simulink model "sampleModel541_pp_difftest"  (R2021a)
settings: Solver=VariableStepAuto  StartTime=0.0  StopTime=10.0  RelTol=1e-3
undefined symbols (not defined in the file): DiscIntNeverNeededParam, Newton, Raphson
libraries: simulink x23, pid_lib x5
settings Model: Creator=user  LastModifiedBy=user

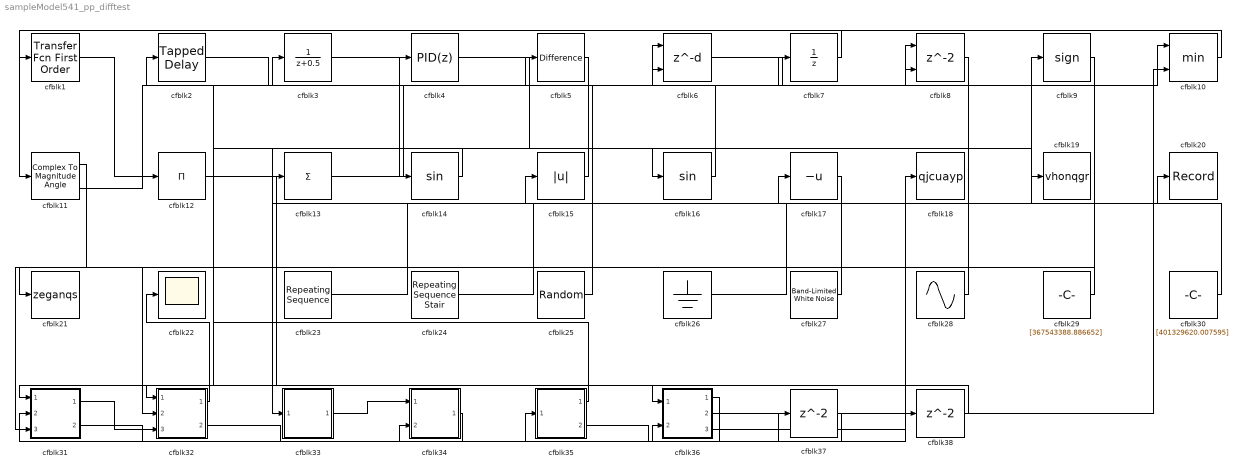
== system sampleModel541_pp_difftest ==
  cfblk1 : simulink/Discrete/Transfer Fcn First Order  PoleZ=0.95  ICPrevOutput=0.0  DoSatur=off
  cfblk10 : MinMax  Inputs=2
  cfblk11 : ComplexToMagnitudeAngle
  cfblk12 : Product  Inputs=*
  cfblk13 : Sum  Inputs=+
  cfblk14 : Trigonometry
  cfblk15 : Abs
  cfblk16 : Trigonometry
  cfblk17 : UnaryMinus
  cfblk18 : ToWorkspace  VariableName=qjcuayp  SaveFormat=Timeseries  SampleTime=-1
  cfblk19 : ToWorkspace  VariableName=vhonqgr  SaveFormat=Timeseries  SampleTime=-1
  cfblk2 : simulink/Discrete/Tapped Delay  vinit=0.0  samptime=-1  NumDelays=1  DelayOrder=Oldest  includeCurrent=off
  cfblk20 : Record  FileSettingsInternal="{\"entries\":[{\"content\":{\"excelSettings\":{\"content\":{},\"type\":\"Streamout.ExcelSettings\"}},\"type\":\"Streamout.FileSettingStorage\",\"uuid\":\"01edc3a3-d80d-4732-8608-4e9d142ed4ab\"}],\"packageUris\":[\"http://schema.mathworks.com/mf0/streamout_blocks/R2020a\"],\"version\":\"1.0\"}"  SignalsInternal="{\"entries\":[{\"content\":{\"signals\":[{\"content\":{\"blockPath\":[\"sampleModel541_pp_difftest/cfblk20\"],\"channel\":[],\"dimensions\":[1],\"domain\":\"samplemodel541_pp_difftest/cfblk20\",\"lineColor\":\"#7e2f8e\",\"plots\":[1],\"port\":1,\"sid\":[],\"signalID\":19,\"signalName\":\"cfblk24\"},\"type\":\"RecordBlkView.Signal\",\"uuid\":\"c9c95548-154d-48a7-8825-4786a1f0d84d\"}]},\"type\":\"RecordBlkView.InputSignals\",\"uuid\":\"a5788f2e-6ff7-4599-b457-e45010491cd0\"}],\"packageUris\":[\"http://schema.mathworks.com/mf0/streamout_blocks/R2020a\"],\"version\":\"1.0\"}"  VisualizationBindings="{\"sparklinesplugin\":{\"info\":[{\"bindingParametersList\":[],\"subplotID\":1}]}}"
  cfblk21 : ToWorkspace  VariableName=zeganqs  SaveFormat=Timeseries  SampleTime=-1
  cfblk22 : Scope
  cfblk23 : simulink/Sources/Repeating Sequence  rep_seq_t=[0 2]  rep_seq_y=[416477790.425688, 725633583.092416]
  cfblk24 : simulink/Sources/Repeating Sequence Stair  OutValues=[-702429095.453026, -136139678.587980]  tsamp=-1  OutMin=[]  OutMax=[]  OutDataTypeStr=double  OutputDataTypeScalingMode=double  OutDataType=fixdt(0,8)  ConRadixGroup=Best Precision: Vector-wise  OutScaling=2^-12
  cfblk25 : RandomNumber  Mean=[-5029.199072]  Variance=[76752.887216]  Seed=[360612598.000000]  SampleTime=0.1
  cfblk26 : Ground
  cfblk27 : simulink/Sources/Band-Limited White Noise  Cov=[8491605814.361879]  Ts=0.1  seed=[7568071354.000000]
  cfblk28 : Sin  Amplitude=[59962648.551395]  Bias=[-800425245.596998]  SampleTime=0
  cfblk29 : Constant  Value=[367543388.886652]  SampleTime=1
  cfblk3 : DiscreteTransferFcn  SampleTime=1
  cfblk30 : Constant  Value=[401329620.007595]  SampleTime=1
  cfblk31 : Subsystem
  cfblk32 : Subsystem
  cfblk33 : Subsystem
  cfblk34 : Subsystem
  cfblk35 : Subsystem
  cfblk36 : Subsystem
  cfblk37 : Delay  SampleTime=1
  cfblk38 : Delay  SampleTime=1
  cfblk4 : pid_lib/PID Controller  Controller=PID  Form=Parallel  TimeDomain=Discrete-time  UseExternalTs=off  SampleTime=1  IntegratorMethod=Forward Euler  FilterMethod=Forward Euler  ControllerParametersSource=internal  P=1  I=1  D=0  UseFilter=on  N=100  TunerSelectOption=Transfer Function Based (PID Tuner App)  InitialConditionSource=internal  InitialConditionForIntegrator=0  InitialConditionForFilter=0  DifferentiatorICPrevScaledInput=0  ExternalReset=none  TrackingMode=off  Kt=1  LimitOutput=off  SatLimitsSource=internal  UpperSaturationLimit=inf  LowerSaturationLimit=-inf  LinearizeAsGain=off  AntiWindupMode=none  Kb=1  POutMin=[]  POutMax=[]  IOutMin=[]  IOutMax=[]  DOutMin=[]  DOutMax=[]  NOutMin=[]  NOutMax=[]  SumOutMin=[]  SumOutMax=[]  SaturationOutMin=[]  SaturationOutMax=[]  PParamMin=[]  PParamMax=[]  IParamMin=[]  IParamMax=[]  DParamMin=[]  DParamMax=[]  NParamMin=[]  NParamMax=[]  KbParamMin=[]  KbParamMax=[]  KtParamMin=[]  KtParamMax=[]  KbOutMin=[]  KbOutMax=[]  KtOutMin=[]  KtOutMax=[]  IntegratorOutMin=[]  IntegratorOutMax=[]  FilterOutMin=[]  FilterOutMax=[]  SumI1OutMin=[]  SumI1OutMax=[]  SumI2OutMin=[]  SumI2OutMax=[]  SumI3OutMin=[]  SumI3OutMax=[]  SumI4OutMin=[]  SumI4OutMax=[]  SumDOutMin=[]  SumDOutMax=[]  DifferentiatorOutMin=[]  DifferentiatorOutMax=[]  FilterDiffOutCoefMin=[]  FilterDiffOutCoefMax=[]  ReciprocalOutMin=[]  ReciprocalOutMax=[]  SumDenOutMin=[]  SumDenOutMax=[]  SumNumOutMin=[]  SumNumOutMax=[]  DivideOutMin=[]  DivideOutMax=[]  UdiffTsProdOutMin=[]  UdiffTsProdOutMax=[]  NTsProdOutMin=[]  NTsProdOutMax=[]  UintegralTsProdOutMin=[]  UintegralTsProdOutMax=[]  UngainTsProdOutMin=[]  UngainTsProdOutMax=[]  IntegratorContinuousStateAttributes=''  IntegratorStateMustResolveToSignalObject=off  IntegratorRTWStateStorageClass=Auto  FilterContinuousStateAttributes=''  FilterStateMustResolveToSignalObject=off  FilterRTWStateStorageClass=Auto  ParallelPVariant=InternalParameters  IdealPVariant=Disabled  IVariant=InternalParameters  DVariant=InternalParameters  IntegratorVariant=Discrete  SatVariant=Disabled  AWVariant=Passthrough  PCopyVariant=Disabled  TRVariant=Disabled  FdbkBlocksVariant=Forward  IdealPFdbkVariant=Disabled  SatFdbkVariant=Disabled  DerivativeFilterVariant=ForwardEulerFilter  NVariant=InternalParameters  NCopyVariant=Disabled  FilterICVariant=InternalICsFilter  IntegratorICVariant=InternalICs  ExternalResetVariant=Disabled  TRSumVariant=Passthrough  SumFdbkVariant=Disabled  SumVariant=Sum_PID  TsampFilterVariant=InternalTs  TsampNgainVariant=Passthrough  TsampIntegralVariant=Passthrough  ExternalSaturationOutDataTypeStr=Inherit: Same as second input
  cfblk5 : simulink/Discrete/Difference  ICPrevInput=0.0  OutMin=[]  OutMax=[]  OutDataTypeStr=Inherit: Inherit via back propagation  OutDataType=fixdt(1, 16)  OutScaling=2^-10  DoSatur=off
  cfblk6 : Delay  DelayLengthSource=Input port  SampleTime=1
      settings: InputPortMap=u0,p1
  cfblk7 : UnitDelay  HasFrameUpgradeWarning=on
  cfblk8 : Delay  ShowEnablePort=on  SampleTime=1
      settings: InputPortMap=u0,e6
  cfblk9 : Signum
  wires:
  cfblk1/1 -> cfblk12/1
  cfblk10/1 -> cfblk11/1
  cfblk23/1 -> cfblk15/1
  cfblk24/1 -> cfblk20/1
  cfblk14/1 -> cfblk32/1(cfblk1)
  cfblk13/1 -> cfblk6/1
  cfblk35/1(cfblk2) -> cfblk2/1
  cfblk6/1 -> cfblk10/1
  cfblk3/1 -> cfblk14/1
  cfblk33/1(cfblk2) -> cfblk34/1(cfblk1)
  cfblk16/1 -> cfblk4/1
  cfblk5/1 -> cfblk33/1(cfblk1)
  cfblk26/1 -> cfblk9/1
  cfblk17/1 -> cfblk32/2(cfblk13)
  cfblk11/1 -> cfblk21/1
  cfblk32/1(cfblk2) -> cfblk22/1
  cfblk28/1 -> cfblk8/1
  cfblk29/1 -> cfblk7/1
  cfblk8/1 -> cfblk16/1
  cfblk12/1 -> cfblk36/1(cfblk1)
  cfblk7/1 -> cfblk1/1
  cfblk36/1(cfblk2) -> cfblk34/2(cfblk8)
  cfblk15/1 -> cfblk3/1
  cfblk27/1 -> cfblk13/1
  cfblk4/1 -> cfblk19/1
  cfblk2/1 -> cfblk6/2
  cfblk25/1 -> cfblk5/1
  cfblk30/1 -> cfblk17/1
  cfblk31/1(cfblk2) -> cfblk32/3(cfblk14)
  cfblk36/2(cfblk15) -> cfblk10/2
  cfblk31/2(cfblk12) -> cfblk35/1(cfblk1)
  cfblk34/1(cfblk2) -> cfblk31/2(cfblk10)
  cfblk9/1 -> cfblk31/3(cfblk11)
  cfblk11/2 -> cfblk8/2
  cfblk36/3(cfblk16) -> cfblk18/1
  cfblk32/2(cfblk15) -> cfblk37/1
  cfblk37/1 -> cfblk36/2(cfblk14)
  cfblk35/2(cfblk14) -> cfblk38/1
  cfblk38/1 -> cfblk31/1(cfblk1)

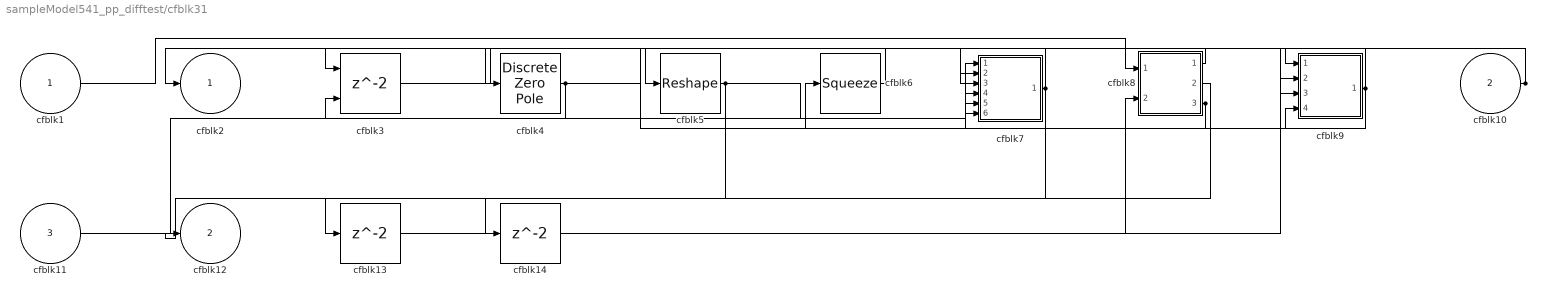
== system sampleModel541_pp_difftest/cfblk31 ==
  cfblk1 : Inport
  cfblk10 : Inport  Port=2
  cfblk11 : Inport  Port=3
  cfblk13 : Delay  SampleTime=1
  cfblk14 : Delay  SampleTime=1
  cfblk3 : Delay  ShowEnablePort=on  SampleTime=1
      settings: InputPortMap=u0,e6
  cfblk4 : DiscreteZeroPole  Poles=[0 0.5]  Gain=1
  cfblk5 : Reshape
  cfblk6 : Squeeze
  cfblk7 : Subsystem
  cfblk8 : Subsystem
  cfblk9 : Subsystem
  cfblk2 : Outport
  cfblk12 : Outport  Port=2
  wires:
  cfblk11/1 -> cfblk7/1(cfblk1)
  cfblk7/1(cfblk2) -> cfblk2/1, cfblk14/1
  cfblk1/1 -> cfblk8/1(cfblk1)
  cfblk8/1(cfblk2) -> cfblk3/1
  cfblk4/1 -> cfblk3/2, cfblk9/3(cfblk15), cfblk9/4(cfblk16)
  cfblk5/1 -> cfblk7/5(cfblk14), cfblk13/1
  cfblk8/2(cfblk14) -> cfblk12/1
  cfblk8/3(cfblk15) -> cfblk6/1, cfblk7/6(cfblk15)
  cfblk9/1(cfblk2) -> cfblk5/1, cfblk7/4(cfblk13)
  cfblk10/1 -> cfblk7/2(cfblk11), cfblk7/3(cfblk12)
  cfblk3/1 -> cfblk9/1(cfblk1)
  cfblk6/1 -> cfblk4/1
  cfblk13/1 -> cfblk8/2(cfblk13)
  cfblk14/1 -> cfblk9/2(cfblk14)

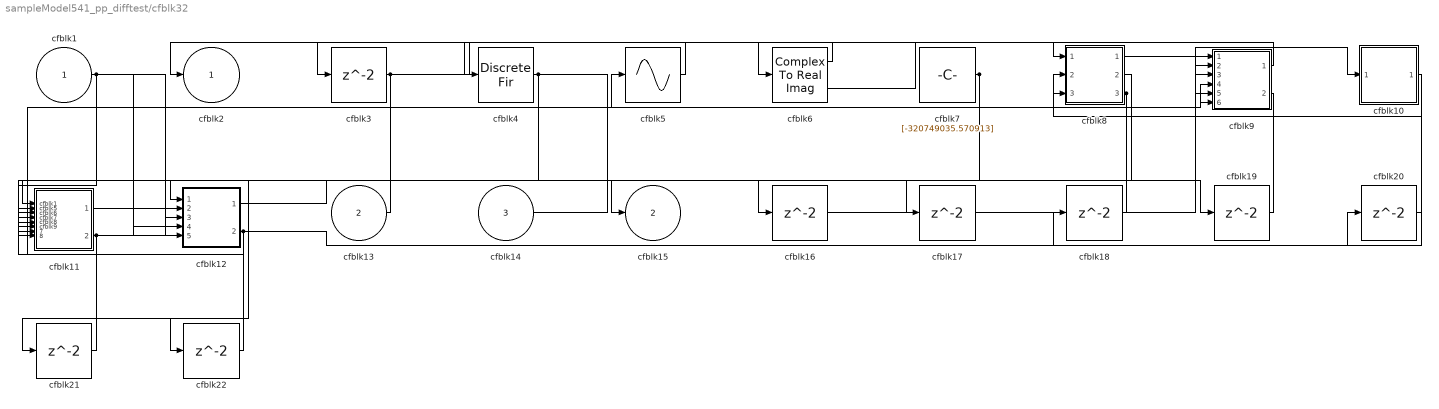
== system sampleModel541_pp_difftest/cfblk32 ==
  cfblk1 : Inport
  cfblk13 : Inport  Port=2
  cfblk14 : Inport  Port=3
  cfblk10 : Subsystem
  cfblk11 : Subsystem
  cfblk12 : Subsystem
  cfblk{3,16..22} (8 alike) : Delay  SampleTime=1
  cfblk4 : DiscreteFir  SampleTime=1
  cfblk5 : Sin  TimeSource=Use external signal  SampleTime=0
  cfblk6 : ComplexToRealImag
  cfblk7 : Constant  Value=[-320749035.570913]  SampleTime=1
  cfblk8 : Subsystem
  cfblk9 : Subsystem
  cfblk2 : Outport
  cfblk15 : Outport  Port=2
  wires:
  cfblk7/1 -> cfblk15/1, cfblk11/2(cfblk5)
  cfblk3/1 -> cfblk6/1, cfblk11/3(cfblk6), cfblk11/5(cfblk8)
  cfblk4/1 -> cfblk11/4(cfblk7), cfblk16/1
  cfblk5/1 -> cfblk2/1
  cfblk11/2(cfblk12) -> cfblk5/1, cfblk8/3(cfblk7)
  cfblk14/1 -> cfblk9/4(cfblk14)
  cfblk12/2(cfblk12) -> cfblk20/1, cfblk21/1
  cfblk1/1 -> cfblk9/6(cfblk16), cfblk12/4(cfblk10), cfblk12/5(cfblk11), cfblk11/8(cfblk11)
  cfblk6/1 -> cfblk4/1
  cfblk6/2 -> cfblk8/1(cfblk1)
  cfblk8/1(cfblk2) -> cfblk10/1(cfblk1)
  cfblk13/1 -> cfblk12/1(cfblk1)
  cfblk9/1(cfblk2) -> cfblk3/1
  cfblk9/2(cfblk17) -> cfblk8/2(cfblk6)
  cfblk8/2(cfblk8) -> cfblk12/2(cfblk8)
  cfblk8/3(cfblk9) -> cfblk12/3(cfblk9), cfblk22/1
  cfblk16/1 -> cfblk9/1(cfblk1)
  cfblk11/1(cfblk2) -> cfblk17/1
  cfblk17/1 -> cfblk9/2(cfblk12)
  cfblk10/1(cfblk2) -> cfblk18/1
  cfblk18/1 -> cfblk11/1(cfblk1)
  cfblk12/1(cfblk2) -> cfblk19/1
  cfblk19/1 -> cfblk9/3(cfblk13)
  cfblk20/1 -> cfblk9/5(cfblk15)
  cfblk21/1 -> cfblk11/7(cfblk10)
  cfblk22/1 -> cfblk11/6(cfblk9)

== system sampleModel541_pp_difftest/cfblk33 ==
  cfblk1 : Inport
  cfblk10 : Delay  SampleTime=1
  cfblk3 : Product  Inputs=*
  cfblk4 : Signum
  cfblk5 : Subsystem
  cfblk6 : Subsystem
  cfblk7 : Subsystem
  cfblk8 : Delay  SampleTime=1
  cfblk9 : Delay  SampleTime=1
  cfblk2 : Outport
  wires:
  cfblk6/1(cfblk2) -> cfblk4/1
  cfblk1/1 -> cfblk2/1
  cfblk3/1 -> cfblk5/2(cfblk8)
  cfblk5/1(cfblk2) -> cfblk6/2(cfblk9)
  cfblk5/2(cfblk9) -> cfblk7/1(cfblk1)
  cfblk4/1 -> cfblk8/1
  cfblk8/1 -> cfblk6/1(cfblk1)
  cfblk7/1(cfblk2) -> cfblk9/1
  cfblk9/1 -> cfblk5/1(cfblk1)
  cfblk7/2(cfblk7) -> cfblk10/1
  cfblk10/1 -> cfblk3/1

== system sampleModel541_pp_difftest/cfblk34 ==
  cfblk1 : Inport
  cfblk8 : Inport  Port=2
  cfblk{9..14} (6 alike) : Delay  SampleTime=1
  cfblk3 : simulink/Discrete/Tapped Delay  vinit=0.0  samptime=-1  NumDelays=1  DelayOrder=Oldest  includeCurrent=off
  cfblk4 : Product
  cfblk5 : Product
  cfblk6 : Sum  Inputs=+-
  cfblk7 : Subsystem
  cfblk2 : Outport
  wires:
  cfblk4/1 -> cfblk3/1, cfblk13/1
  cfblk8/1 -> cfblk6/1
  cfblk1/1 -> cfblk2/1, cfblk7/4(cfblk14)
  cfblk5/1 -> cfblk9/1, cfblk10/1, cfblk11/1
  cfblk7/1(cfblk2) -> cfblk6/2
  cfblk3/1 -> cfblk5/1, cfblk12/1
  cfblk6/1 -> cfblk4/2, cfblk14/1
  cfblk7/2(cfblk17) -> cfblk5/2
  cfblk9/1 -> cfblk4/1
  cfblk10/1 -> cfblk7/2(cfblk12)
  cfblk11/1 -> cfblk7/3(cfblk13)
  cfblk12/1 -> cfblk7/1(cfblk1)
  cfblk13/1 -> cfblk7/5(cfblk15)
  cfblk14/1 -> cfblk7/6(cfblk16)

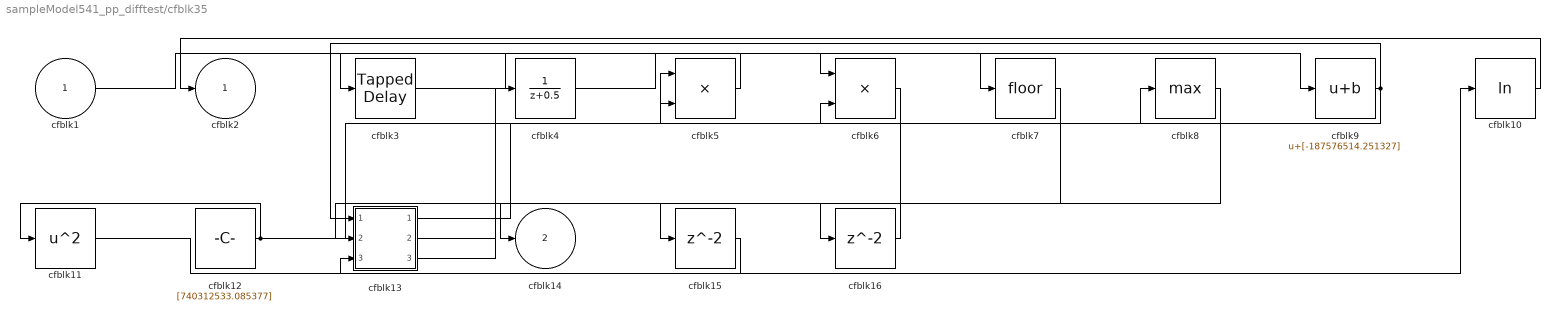
== system sampleModel541_pp_difftest/cfblk35 ==
  cfblk1 : Inport
  cfblk10 : Math  Operator=log  SaturateOnIntegerOverflow=on
  cfblk11 : Math  Operator=square  SaturateOnIntegerOverflow=on
  cfblk12 : Constant  Value=[740312533.085377]  SampleTime=1
  cfblk13 : Subsystem
  cfblk15 : Delay  SampleTime=1
  cfblk16 : Delay  SampleTime=1
  cfblk3 : simulink/Discrete/Tapped Delay  vinit=0.0  samptime=-1  NumDelays=1  DelayOrder=Oldest  includeCurrent=off
  cfblk4 : DiscreteTransferFcn  SampleTime=1
  cfblk5 : Product  Inputs=**
  cfblk6 : Product  Inputs=**
  cfblk7 : Rounding
  cfblk8 : MinMax  Function=max
  cfblk9 : Bias  Bias=[-187576514.251327]
  cfblk2 : Outport
  cfblk14 : Outport  Port=2
  wires:
  cfblk5/1 -> cfblk3/1
  cfblk12/1 -> cfblk5/1, cfblk11/1
  cfblk9/1 -> cfblk13/1(cfblk1), cfblk6/2
  cfblk11/1 -> cfblk10/1
  cfblk3/1 -> cfblk7/1
  cfblk13/1(cfblk2) -> cfblk5/2
  cfblk10/1 -> cfblk2/1
  cfblk1/1 -> cfblk9/1
  cfblk8/1 -> cfblk14/1
  cfblk4/1 -> cfblk6/1
  cfblk13/2(cfblk12) -> cfblk8/1
  cfblk13/3(cfblk13) -> cfblk4/1
  cfblk7/1 -> cfblk15/1
  cfblk15/1 -> cfblk13/3(cfblk11)
  cfblk6/1 -> cfblk16/1
  cfblk16/1 -> cfblk13/2(cfblk10)

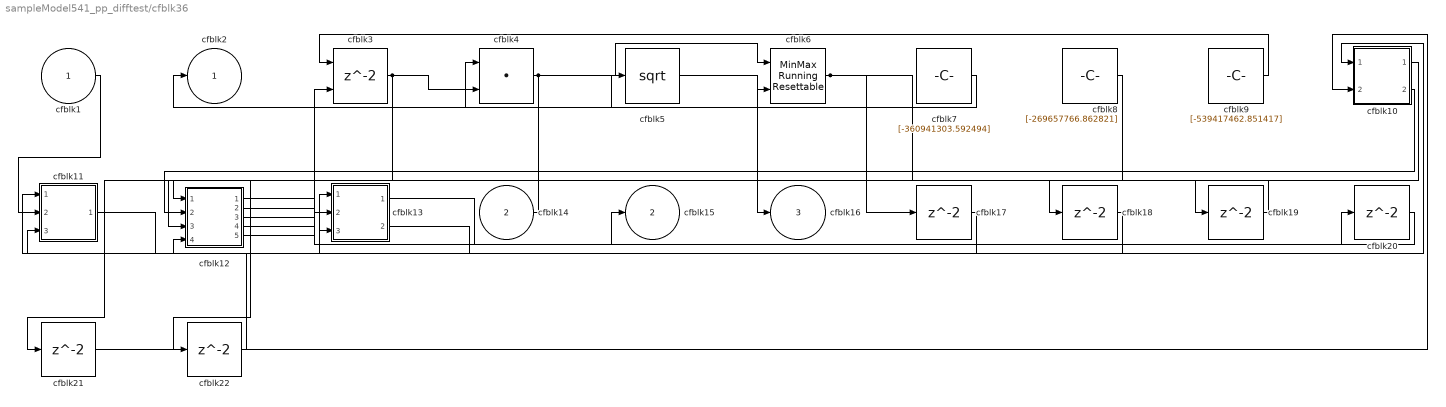
== system sampleModel541_pp_difftest/cfblk36 ==
  cfblk1 : Inport
  cfblk14 : Inport  Port=2
  cfblk10 : Subsystem
  cfblk11 : Subsystem
  cfblk12 : Subsystem
  cfblk13 : Subsystem
  cfblk{17..22} (6 alike) : Delay  SampleTime=1
  cfblk3 : Delay  ShowEnablePort=on  SampleTime=1
      settings: InputPortMap=u0,e6
  cfblk4 : DotProduct  InputSameDT=on  OutDataTypeStr=Inherit: Inherit via internal rule
  cfblk5 : Sqrt  SaturateOnIntegerOverflow=on
  cfblk6 : simulink/Math Operations/MinMax Running Resettable  Function=min  vinit=0.0
  cfblk7 : Constant  Value=[-360941303.592494]  SampleTime=1
  cfblk8 : Constant  Value=[-269657766.862821]  SampleTime=1
  cfblk9 : Constant  Value=[-539417462.851417]  SampleTime=1
  cfblk2 : Outport
  cfblk15 : Outport  Port=2
  cfblk16 : Outport  Port=3
  wires:
  cfblk10/1(cfblk2) -> cfblk12/1(cfblk1)
  cfblk4/1 -> cfblk6/1, cfblk21/1
  cfblk7/1 -> cfblk5/1
  cfblk10/2(cfblk8) -> cfblk12/2(cfblk8)
  cfblk3/1 -> cfblk4/2, cfblk22/1
  cfblk14/1 -> cfblk2/1
  cfblk9/1 -> cfblk3/1
  cfblk8/1 -> cfblk12/3(cfblk9)
  cfblk5/1 -> cfblk16/1
  cfblk11/1(cfblk2) -> cfblk13/1(cfblk1)
  cfblk13/1(cfblk2) -> cfblk15/1
  cfblk6/1 -> cfblk17/1, cfblk18/1
  cfblk12/1(cfblk2) -> cfblk6/2
  cfblk1/1 -> cfblk11/2(cfblk6)
  cfblk13/2(cfblk16) -> cfblk10/1(cfblk1)
  cfblk12/4(cfblk13) -> cfblk4/1
  cfblk12/5(cfblk14) -> cfblk3/2
  cfblk17/1 -> cfblk12/4(cfblk10)
  cfblk18/1 -> cfblk11/3(cfblk7)
  cfblk12/2(cfblk11) -> cfblk19/1
  cfblk19/1 -> cfblk13/2(cfblk14)
  cfblk12/3(cfblk12) -> cfblk20/1
  cfblk20/1 -> cfblk13/3(cfblk15)
  cfblk21/1 -> cfblk10/2(cfblk7)
  cfblk22/1 -> cfblk11/1(cfblk1)

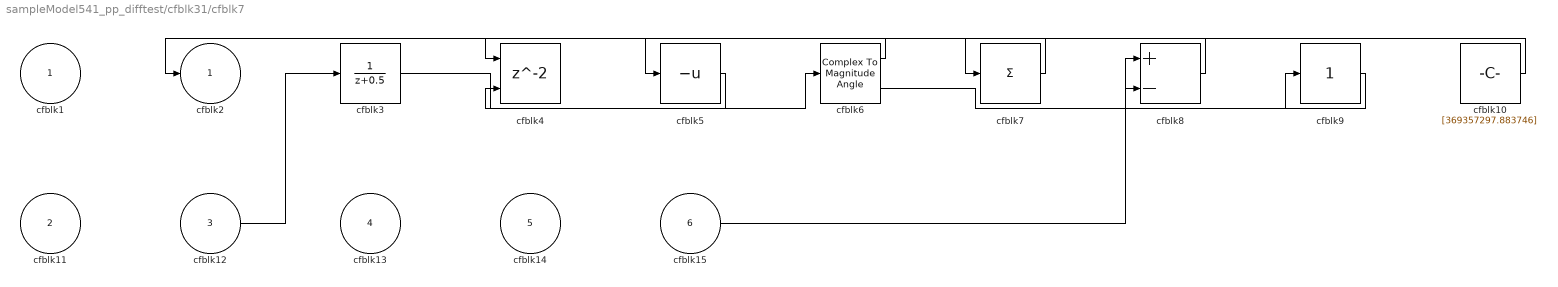
== system sampleModel541_pp_difftest/cfblk31/cfblk7 ==
  cfblk1 : Inport
  cfblk11 : Inport  Port=2
  cfblk12 : Inport  Port=3
  cfblk13 : Inport  Port=4
  cfblk14 : Inport  Port=5
  cfblk15 : Inport  Port=6
  cfblk10 : Constant  Value=[369357297.883746]  SampleTime=1
  cfblk3 : DiscreteTransferFcn  SampleTime=1
  cfblk4 : Delay  ShowEnablePort=on  SampleTime=1
      settings: InputPortMap=u0,e6
  cfblk5 : UnaryMinus
  cfblk6 : ComplexToMagnitudeAngle
  cfblk7 : Sum  Inputs=+
  cfblk8 : Sum  Inputs=+-
  cfblk9 : simulink/Math Operations/Slider Gain  gain=1  low=0  high=2
  cfblk2 : Outport
  wires:
  cfblk6/1 -> cfblk2/1
  cfblk6/2 -> cfblk9/1
  cfblk8/1 -> cfblk7/1
  cfblk7/1 -> cfblk5/1
  cfblk3/1 -> cfblk6/1
  cfblk10/1 -> cfblk4/1
  cfblk15/1 -> cfblk8/1
  cfblk12/1 -> cfblk3/1
  cfblk5/1 -> cfblk4/2
  cfblk9/1 -> cfblk8/2

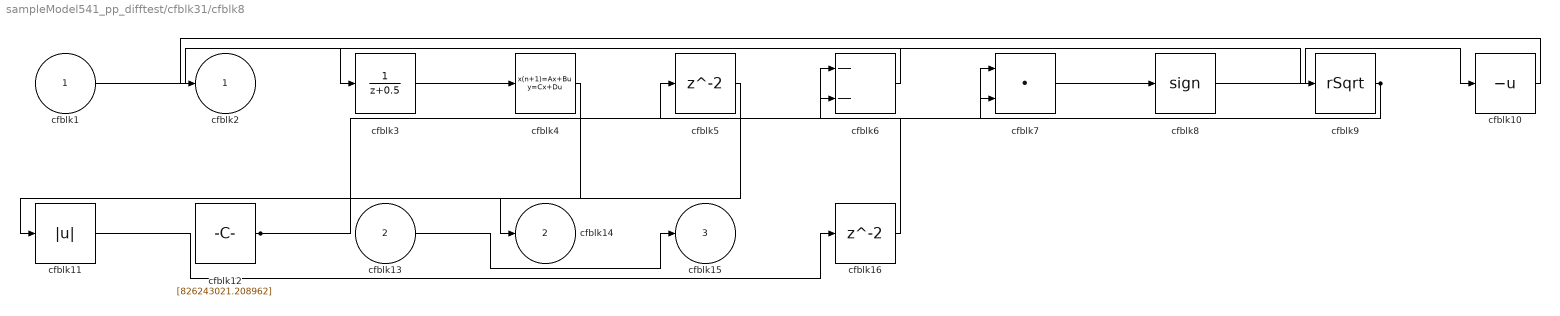
== system sampleModel541_pp_difftest/cfblk31/cfblk8 ==
  cfblk1 : Inport
  cfblk13 : Inport  Port=2
  cfblk10 : UnaryMinus
  cfblk11 : Abs
  cfblk12 : Constant  Value=[826243021.208962]  SampleTime=1
  cfblk16 : Delay  SampleTime=1
  cfblk3 : DiscreteTransferFcn  SampleTime=1
  cfblk4 : DiscreteStateSpace
  cfblk5 : Delay  SampleTime=1
  cfblk6 : Sum  Inputs=--
  cfblk7 : DotProduct  InputSameDT=on  OutDataTypeStr=Inherit: Inherit via internal rule
  cfblk8 : Signum
  cfblk9 : Sqrt  Operator=rSqrt  AlgorithmType=Newton-Raphson  SaturateOnIntegerOverflow=on
  cfblk2 : Outport
  cfblk14 : Outport  Port=2
  cfblk15 : Outport  Port=3
  wires:
  cfblk8/1 -> cfblk10/1
  cfblk4/1 -> cfblk14/1
  cfblk3/1 -> cfblk4/1
  cfblk9/1 -> cfblk6/1, cfblk7/2
  cfblk1/1 -> cfblk9/1
  cfblk12/1 -> cfblk6/2, cfblk7/1
  cfblk13/1 -> cfblk15/1
  cfblk7/1 -> cfblk8/1
  cfblk6/1 -> cfblk3/1
  cfblk5/1 -> cfblk11/1
  cfblk10/1 -> cfblk2/1
  cfblk11/1 -> cfblk16/1
  cfblk16/1 -> cfblk5/1

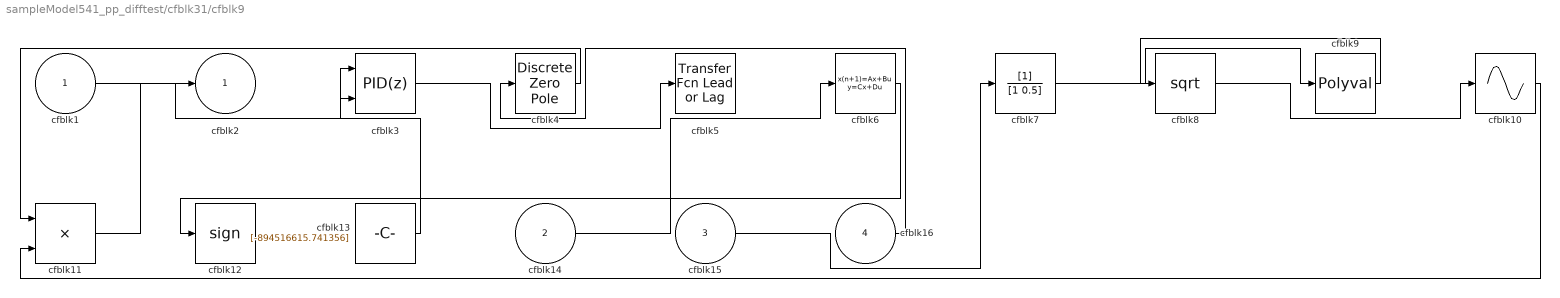
== system sampleModel541_pp_difftest/cfblk31/cfblk9 ==
  cfblk1 : Inport
  cfblk14 : Inport  Port=2
  cfblk15 : Inport  Port=3
  cfblk16 : Inport  Port=4
  cfblk10 : Sin  TimeSource=Use external signal  SampleTime=0
  cfblk11 : Product  Inputs=**
  cfblk12 : Signum
  cfblk13 : Constant  Value=[-894516615.741356]  SampleTime=1
  cfblk3 : pid_lib/PID Controller (2DOF)  Controller=PID  Form=Parallel  TimeDomain=Discrete-time  UseExternalTs=off  SampleTime=1  IntegratorMethod=Forward Euler  FilterMethod=Forward Euler  ControllerParametersSource=internal  P=1  I=1  D=0  UseFilter=on  N=100  b=1  c=1  TunerSelectOption=Transfer Function Based (PID Tuner App)  InitialConditionSource=internal  InitialConditionForIntegrator=0  InitialConditionForFilter=0  DifferentiatorICPrevScaledInput=0  ExternalReset=none  TrackingMode=off  Kt=1  LimitOutput=off  SatLimitsSource=internal  UpperSaturationLimit=inf  LowerSaturationLimit=-inf  LinearizeAsGain=off  AntiWindupMode=none  Kb=1  POutMin=[]  POutMax=[]  IOutMin=[]  IOutMax=[]  DOutMin=[]  DOutMax=[]  NOutMin=[]  NOutMax=[]  bOutMin=[]  bOutMax=[]  cOutMin=[]  cOutMax=[]  SumOutMin=[]  SumOutMax=[]  SaturationOutMin=[]  SaturationOutMax=[]  PParamMin=[]  PParamMax=[]  IParamMin=[]  IParamMax=[]  DParamMin=[]  DParamMax=[]  NParamMin=[]  NParamMax=[]  bParamMin=[]  bParamMax=[]  cParamMin=[]  cParamMax=[]  KbParamMin=[]  KbParamMax=[]  KtParamMin=[]  KtParamMax=[]  KbOutMin=[]  KbOutMax=[]  KtOutMin=[]  KtOutMax=[]  IntegratorOutMin=[]  IntegratorOutMax=[]  FilterOutMin=[]  FilterOutMax=[]  SumI1OutMin=[]  SumI1OutMax=[]  SumI2OutMin=[]  SumI2OutMax=[]  SumI3OutMin=[]  SumI3OutMax=[]  SumI4OutMin=[]  SumI4OutMax=[]  SumDOutMin=[]  SumDOutMax=[]  Sum1OutMin=[]  Sum1OutMax=[]  Sum2OutMin=[]  Sum2OutMax=[]  Sum3OutMin=[]  Sum3OutMax=[]  DifferentiatorOutMin=[]  DifferentiatorOutMax=[]  FilterDiffOutCoefMin=[]  FilterDiffOutCoefMax=[]  ReciprocalOutMin=[]  ReciprocalOutMax=[]  SumDenOutMin=[]  SumDenOutMax=[]  SumNumOutMin=[]  SumNumOutMax=[]  DivideOutMin=[]  DivideOutMax=[]  UdiffTsProdOutMin=[]  UdiffTsProdOutMax=[]  NTsProdOutMin=[]  NTsProdOutMax=[]  UintegralTsProdOutMin=[]  UintegralTsProdOutMax=[]  UngainTsProdOutMin=[]  UngainTsProdOutMax=[]  IntegratorContinuousStateAttributes=''  IntegratorStateMustResolveToSignalObject=off  IntegratorRTWStateStorageClass=Auto  FilterContinuousStateAttributes=''  FilterStateMustResolveToSignalObject=off  FilterRTWStateStorageClass=Auto  ParallelPVariant=InternalParameters  IdealPVariant=Disabled  IVariant=InternalParameters  DVariant=InternalParameters  bVariant=InternalParameters  cVariant=InternalParameters  IntegratorVariant=Discrete  SatVariant=Disabled  AWVariant=Passthrough  PCopyVariant=Disabled  TRVariant=Disabled  FdbkBlocksVariant=Forward  IdealPFdbkVariant=Disabled  SatFdbkVariant=Disabled  DerivativeFilterVariant=ForwardEulerFilter  NVariant=InternalParameters  NCopyVariant=Disabled  FilterICVariant=InternalICsFilter  IntegratorICVariant=InternalICs  ExternalResetVariant=Disabled  TRSumVariant=Passthrough  SumFdbkVariant=Disabled  SumVariant=Sum_PID  TsampFilterVariant=InternalTs  TsampNgainVariant=Passthrough  TsampIntegralVariant=Passthrough  ExternalSaturationOutDataTypeStr=Inherit: Same as second input
      settings: SourceProductBaseCode=SL
  cfblk4 : DiscreteZeroPole  Poles=[0 0.5]  Gain=1
  cfblk5 : simulink/Discrete/Transfer Fcn Lead or Lag  PoleZ=0.95  ZeroZ=0.75  ICPrevOutput=0.0  ICPrevInput=0.0  DoSatur=off
      settings: SourceProductBaseCode=SL
  cfblk6 : DiscreteStateSpace
  cfblk7 : DiscreteFilter  SampleTime=1
  cfblk8 : Sqrt  SaturateOnIntegerOverflow=on
  cfblk9 : Polyval  Coefs=[ +2.081618890e-019, -1.441693666e-014, +4.719686976e-010, -8.536869453e-006, +1.621573104e-001, -8.087801117e+001 ]
  cfblk2 : Outport
  wires:
  cfblk6/1 -> cfblk12/1
  cfblk11/1 -> cfblk2/1
  cfblk13/1 -> cfblk3/1
  cfblk14/1 -> cfblk6/1
  cfblk4/1 -> cfblk11/1
  cfblk7/1 -> cfblk9/1
  cfblk15/1 -> cfblk7/1
  cfblk8/1 -> cfblk10/1
  cfblk10/1 -> cfblk11/2
  cfblk9/1 -> cfblk8/1
  cfblk1/1 -> cfblk3/2
  cfblk16/1 -> cfblk4/1
  cfblk3/1 -> cfblk5/1

== system sampleModel541_pp_difftest/cfblk32/cfblk10 ==
  cfblk1 : Inport
  cfblk3 : DiscreteFir  SampleTime=1
  cfblk4 : Product  Inputs=*
  cfblk5 : Squeeze
  cfblk6 : Product  Inputs=**
  cfblk7 : Math  SaturateOnIntegerOverflow=on
  cfblk2 : Outport
  wires:
  cfblk6/1 -> cfblk2/1
  cfblk3/1 -> cfblk6/1
  cfblk1/1 -> cfblk4/1
  cfblk7/1 -> cfblk5/1
  cfblk4/1 -> cfblk7/1, cfblk3/1
  cfblk5/1 -> cfblk6/2

== system sampleModel541_pp_difftest/cfblk32/cfblk11 ==
  cfblk1 : Inport
  cfblk5 : Inport  Port=2
  cfblk6 : Inport  Port=3
  cfblk7 : Inport  Port=4
  cfblk8 : Inport  Port=5
  cfblk9 : Inport  Port=6
  cfblk10 : Inport  Port=7
  cfblk11 : Inport  Port=8
  cfblk3 : simulink/Discrete/Difference  ICPrevInput=0.0  OutMin=[]  OutMax=[]  OutDataTypeStr=Inherit: Inherit via back propagation  OutDataType=fixdt(1, 16)  OutScaling=2^-10  DoSatur=off
  cfblk4 : Polyval  Coefs=[ +2.081618890e-019, -1.441693666e-014, +4.719686976e-010, -8.536869453e-006, +1.621573104e-001, -8.087801117e+001 ]
  cfblk2 : Outport
  cfblk12 : Outport  Port=2
  wires:
  cfblk9/1 -> cfblk2/1
  cfblk3/1 -> cfblk12/1
  cfblk7/1 -> cfblk4/1
  cfblk4/1 -> cfblk3/1

== system sampleModel541_pp_difftest/cfblk32/cfblk12 ==
  cfblk1 : Inport
  cfblk8 : Inport  Port=2
  cfblk9 : Inport  Port=3
  cfblk10 : Inport  Port=4
  cfblk11 : Inport  Port=5
  cfblk3 : DiscreteTransferFcn  SampleTime=1
  cfblk4 : DiscreteTransferFcn  SampleTime=1
  cfblk5 : ComplexToRealImag
  cfblk6 : Abs
  cfblk7 : Sum  Inputs=+
  cfblk2 : Outport
  cfblk12 : Outport  Port=2
  wires:
  cfblk1/1 -> cfblk7/1
  cfblk7/1 -> cfblk12/1
  cfblk9/1 -> cfblk5/1
  cfblk3/1 -> cfblk2/1
  cfblk5/1 -> cfblk3/1
  cfblk5/2 -> cfblk6/1
  cfblk10/1 -> cfblk4/1

== system sampleModel541_pp_difftest/cfblk32/cfblk8 ==
  cfblk1 : Inport
  cfblk6 : Inport  Port=2
  cfblk7 : Inport  Port=3
  cfblk10 : Delay  SampleTime=1
  cfblk3 : DiscreteFilter  SampleTime=1
  cfblk4 : DiscreteZeroPole  Poles=[0 0.5]  Gain=1
  cfblk5 : Product
  cfblk2 : Outport
  cfblk8 : Outport  Port=2
  cfblk9 : Outport  Port=3
  wires:
  cfblk6/1 -> cfblk8/1
  cfblk1/1 -> cfblk9/1
  cfblk5/1 -> cfblk2/1, cfblk10/1
  cfblk3/1 -> cfblk4/1
  cfblk4/1 -> cfblk5/1
  cfblk7/1 -> cfblk5/2
  cfblk10/1 -> cfblk3/1

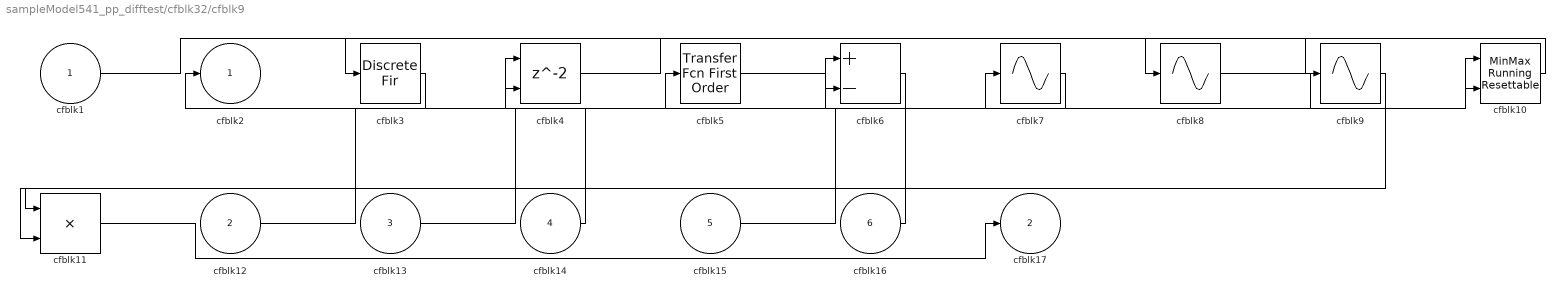
== system sampleModel541_pp_difftest/cfblk32/cfblk9 ==
  cfblk1 : Inport
  cfblk12 : Inport  Port=2
  cfblk13 : Inport  Port=3
  cfblk14 : Inport  Port=4
  cfblk15 : Inport  Port=5
  cfblk16 : Inport  Port=6
  cfblk10 : simulink/Math Operations/MinMax Running Resettable  Function=min  vinit=0.0
  cfblk11 : Product
  cfblk3 : DiscreteFir  SampleTime=1
  cfblk4 : Delay  ShowEnablePort=on  SampleTime=1
      settings: InputPortMap=u0,e6
  cfblk5 : simulink/Discrete/Transfer Fcn First Order  PoleZ=0.95  ICPrevOutput=0.0  DoSatur=off
  cfblk6 : Sum  Inputs=+-
  cfblk7 : Sin  TimeSource=Use external signal  SampleTime=0
  cfblk8 : Sin  TimeSource=Use external signal  SampleTime=0
  cfblk9 : Sin  TimeSource=Use external signal  SampleTime=0
  cfblk2 : Outport
  cfblk17 : Outport  Port=2
  wires:
  cfblk16/1 -> cfblk5/1
  cfblk11/1 -> cfblk17/1
  cfblk10/1 -> cfblk3/1
  cfblk6/1 -> cfblk11/1
  cfblk15/1 -> cfblk10/1
  cfblk9/1 -> cfblk11/2
  cfblk4/1 -> cfblk8/1
  cfblk8/1 -> cfblk10/2
  cfblk14/1 -> cfblk4/1
  cfblk3/1 -> cfblk2/1
  cfblk1/1 -> cfblk9/1
  cfblk13/1 -> cfblk7/1
  cfblk12/1 -> cfblk6/1
  cfblk7/1 -> cfblk4/2
  cfblk5/1 -> cfblk6/2

== system sampleModel541_pp_difftest/cfblk33/cfblk5 ==
  cfblk1 : Inport
  cfblk8 : Inport  Port=2
  cfblk3 : UnitDelay  HasFrameUpgradeWarning=on
  cfblk4 : pid_lib/PID Controller  Controller=PID  Form=Parallel  TimeDomain=Discrete-time  UseExternalTs=off  SampleTime=1  IntegratorMethod=Forward Euler  FilterMethod=Forward Euler  ControllerParametersSource=internal  P=1  I=1  D=0  UseFilter=on  N=100  TunerSelectOption=Transfer Function Based (PID Tuner App)  InitialConditionSource=internal  InitialConditionForIntegrator=0  InitialConditionForFilter=0  DifferentiatorICPrevScaledInput=0  ExternalReset=none  TrackingMode=off  Kt=1  LimitOutput=off  SatLimitsSource=internal  UpperSaturationLimit=inf  LowerSaturationLimit=-inf  LinearizeAsGain=off  AntiWindupMode=none  Kb=1  POutMin=[]  POutMax=[]  IOutMin=[]  IOutMax=[]  DOutMin=[]  DOutMax=[]  NOutMin=[]  NOutMax=[]  SumOutMin=[]  SumOutMax=[]  SaturationOutMin=[]  SaturationOutMax=[]  PParamMin=[]  PParamMax=[]  IParamMin=[]  IParamMax=[]  DParamMin=[]  DParamMax=[]  NParamMin=[]  NParamMax=[]  KbParamMin=[]  KbParamMax=[]  KtParamMin=[]  KtParamMax=[]  KbOutMin=[]  KbOutMax=[]  KtOutMin=[]  KtOutMax=[]  IntegratorOutMin=[]  IntegratorOutMax=[]  FilterOutMin=[]  FilterOutMax=[]  SumI1OutMin=[]  SumI1OutMax=[]  SumI2OutMin=[]  SumI2OutMax=[]  SumI3OutMin=[]  SumI3OutMax=[]  SumI4OutMin=[]  SumI4OutMax=[]  SumDOutMin=[]  SumDOutMax=[]  DifferentiatorOutMin=[]  DifferentiatorOutMax=[]  FilterDiffOutCoefMin=[]  FilterDiffOutCoefMax=[]  ReciprocalOutMin=[]  ReciprocalOutMax=[]  SumDenOutMin=[]  SumDenOutMax=[]  SumNumOutMin=[]  SumNumOutMax=[]  DivideOutMin=[]  DivideOutMax=[]  UdiffTsProdOutMin=[]  UdiffTsProdOutMax=[]  NTsProdOutMin=[]  NTsProdOutMax=[]  UintegralTsProdOutMin=[]  UintegralTsProdOutMax=[]  UngainTsProdOutMin=[]  UngainTsProdOutMax=[]  IntegratorContinuousStateAttributes=''  IntegratorStateMustResolveToSignalObject=off  IntegratorRTWStateStorageClass=Auto  FilterContinuousStateAttributes=''  FilterStateMustResolveToSignalObject=off  FilterRTWStateStorageClass=Auto  ParallelPVariant=InternalParameters  IdealPVariant=Disabled  IVariant=InternalParameters  DVariant=InternalParameters  IntegratorVariant=Discrete  SatVariant=Disabled  AWVariant=Passthrough  PCopyVariant=Disabled  TRVariant=Disabled  FdbkBlocksVariant=Forward  IdealPFdbkVariant=Disabled  SatFdbkVariant=Disabled  DerivativeFilterVariant=ForwardEulerFilter  NVariant=InternalParameters  NCopyVariant=Disabled  FilterICVariant=InternalICsFilter  IntegratorICVariant=InternalICs  ExternalResetVariant=Disabled  TRSumVariant=Passthrough  SumFdbkVariant=Disabled  SumVariant=Sum_PID  TsampFilterVariant=InternalTs  TsampNgainVariant=Passthrough  TsampIntegralVariant=Passthrough  ExternalSaturationOutDataTypeStr=Inherit: Same as second input
  cfblk5 : pid_lib/PID Controller  Controller=PID  Form=Parallel  TimeDomain=Discrete-time  UseExternalTs=off  SampleTime=1  IntegratorMethod=Forward Euler  FilterMethod=Forward Euler  ControllerParametersSource=internal  P=1  I=1  D=0  UseFilter=on  N=100  TunerSelectOption=Transfer Function Based (PID Tuner App)  InitialConditionSource=internal  InitialConditionForIntegrator=0  InitialConditionForFilter=0  DifferentiatorICPrevScaledInput=0  ExternalReset=none  TrackingMode=off  Kt=1  LimitOutput=off  SatLimitsSource=internal  UpperSaturationLimit=inf  LowerSaturationLimit=-inf  LinearizeAsGain=off  AntiWindupMode=none  Kb=1  POutMin=[]  POutMax=[]  IOutMin=[]  IOutMax=[]  DOutMin=[]  DOutMax=[]  NOutMin=[]  NOutMax=[]  SumOutMin=[]  SumOutMax=[]  SaturationOutMin=[]  SaturationOutMax=[]  PParamMin=[]  PParamMax=[]  IParamMin=[]  IParamMax=[]  DParamMin=[]  DParamMax=[]  NParamMin=[]  NParamMax=[]  KbParamMin=[]  KbParamMax=[]  KtParamMin=[]  KtParamMax=[]  KbOutMin=[]  KbOutMax=[]  KtOutMin=[]  KtOutMax=[]  IntegratorOutMin=[]  IntegratorOutMax=[]  FilterOutMin=[]  FilterOutMax=[]  SumI1OutMin=[]  SumI1OutMax=[]  SumI2OutMin=[]  SumI2OutMax=[]  SumI3OutMin=[]  SumI3OutMax=[]  SumI4OutMin=[]  SumI4OutMax=[]  SumDOutMin=[]  SumDOutMax=[]  DifferentiatorOutMin=[]  DifferentiatorOutMax=[]  FilterDiffOutCoefMin=[]  FilterDiffOutCoefMax=[]  ReciprocalOutMin=[]  ReciprocalOutMax=[]  SumDenOutMin=[]  SumDenOutMax=[]  SumNumOutMin=[]  SumNumOutMax=[]  DivideOutMin=[]  DivideOutMax=[]  UdiffTsProdOutMin=[]  UdiffTsProdOutMax=[]  NTsProdOutMin=[]  NTsProdOutMax=[]  UintegralTsProdOutMin=[]  UintegralTsProdOutMax=[]  UngainTsProdOutMin=[]  UngainTsProdOutMax=[]  IntegratorContinuousStateAttributes=''  IntegratorStateMustResolveToSignalObject=off  IntegratorRTWStateStorageClass=Auto  FilterContinuousStateAttributes=''  FilterStateMustResolveToSignalObject=off  FilterRTWStateStorageClass=Auto  ParallelPVariant=InternalParameters  IdealPVariant=Disabled  IVariant=InternalParameters  DVariant=InternalParameters  IntegratorVariant=Discrete  SatVariant=Disabled  AWVariant=Passthrough  PCopyVariant=Disabled  TRVariant=Disabled  FdbkBlocksVariant=Forward  IdealPFdbkVariant=Disabled  SatFdbkVariant=Disabled  DerivativeFilterVariant=ForwardEulerFilter  NVariant=InternalParameters  NCopyVariant=Disabled  FilterICVariant=InternalICsFilter  IntegratorICVariant=InternalICs  ExternalResetVariant=Disabled  TRSumVariant=Passthrough  SumFdbkVariant=Disabled  SumVariant=Sum_PID  TsampFilterVariant=InternalTs  TsampNgainVariant=Passthrough  TsampIntegralVariant=Passthrough  ExternalSaturationOutDataTypeStr=Inherit: Same as second input
  cfblk6 : ComplexToMagnitudeAngle
  cfblk7 : Constant  Value=[-297125752.885891]  SampleTime=1
  cfblk2 : Outport
  cfblk9 : Outport  Port=2
  wires:
  cfblk6/1 -> cfblk4/1
  cfblk1/1 -> cfblk3/1
  cfblk7/1 -> cfblk6/1
  cfblk6/2 -> cfblk2/1
  cfblk8/1 -> cfblk5/1
  cfblk4/1 -> cfblk9/1

== system sampleModel541_pp_difftest/cfblk33/cfblk6 ==
  cfblk1 : Inport
  cfblk9 : Inport  Port=2
  cfblk10 : Delay  SampleTime=1
  cfblk3 : DiscreteTransferFcn  SampleTime=1
  cfblk4 : simulink/Discrete/Transfer Fcn Real Zero  ZeroZ=0.75  ICPrevInput=0.0  DoSatur=off
      settings: SourceProductBaseCode=SL
  cfblk5 : MinMax  Function=max  Inputs=3
  cfblk6 : Product  Inputs=**
  cfblk7 : Trigonometry
  cfblk8 : Trigonometry
  cfblk2 : Outport
  wires:
  cfblk4/1 -> cfblk5/3, cfblk10/1
  cfblk6/1 -> cfblk4/1
  cfblk3/1 -> cfblk6/2
  cfblk9/1 -> cfblk7/1
  cfblk7/1 -> cfblk5/1
  cfblk1/1 -> cfblk5/2, cfblk3/1
  cfblk5/1 -> cfblk8/1
  cfblk8/1 -> cfblk2/1
  cfblk10/1 -> cfblk6/1

== system sampleModel541_pp_difftest/cfblk33/cfblk7 ==
  cfblk1 : Inport
  cfblk3 : Math  Operator=transpose  SaturateOnIntegerOverflow=on
  cfblk4 : Assignment  DiagnosticForDimensions=Warning  IndexOptions=Index vector (dialog)  Indices=1  OutputSizes=1
  cfblk5 : MinMax
  cfblk6 : Constant  Value=[668466041.564327]  SampleTime=1
  cfblk2 : Outport
  cfblk7 : Outport  Port=2
  cfblk8 : Outport  Port=3
  cfblk9 : Outport  Port=4
  wires:
  cfblk3/1 -> cfblk5/1, cfblk7/1
  cfblk6/1 -> cfblk9/1
  cfblk1/1 -> cfblk3/1
  cfblk5/1 -> cfblk8/1, cfblk4/1, cfblk4/2
  cfblk4/1 -> cfblk2/1

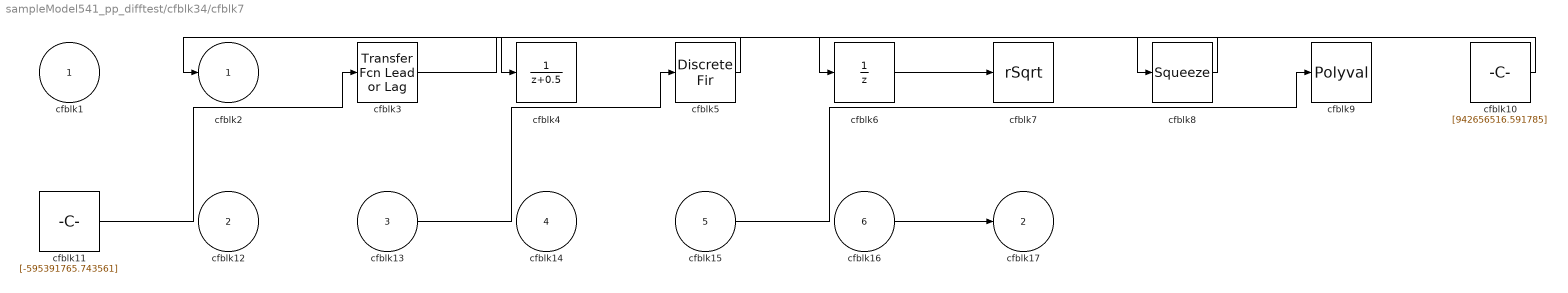
== system sampleModel541_pp_difftest/cfblk34/cfblk7 ==
  cfblk1 : Inport
  cfblk12 : Inport  Port=2
  cfblk13 : Inport  Port=3
  cfblk14 : Inport  Port=4
  cfblk15 : Inport  Port=5
  cfblk16 : Inport  Port=6
  cfblk10 : Constant  Value=[942656516.591785]  SampleTime=1
  cfblk11 : Constant  Value=[-595391765.743561]  SampleTime=1
  cfblk3 : simulink/Discrete/Transfer Fcn Lead or Lag  PoleZ=0.95  ZeroZ=0.75  ICPrevOutput=0.0  ICPrevInput=0.0  DoSatur=off
      settings: SourceProductBaseCode=SL
  cfblk4 : DiscreteTransferFcn  SampleTime=1
  cfblk5 : DiscreteFir  SampleTime=1
  cfblk6 : UnitDelay  HasFrameUpgradeWarning=on
  cfblk7 : Sqrt  Operator=rSqrt  AlgorithmType=Newton-Raphson  SaturateOnIntegerOverflow=on
  cfblk8 : Squeeze
  cfblk9 : Polyval  Coefs=[ +2.081618890e-019, -1.441693666e-014, +4.719686976e-010, -8.536869453e-006, +1.621573104e-001, -8.087801117e+001 ]
  cfblk2 : Outport
  cfblk17 : Outport  Port=2
  wires:
  cfblk16/1 -> cfblk17/1
  cfblk11/1 -> cfblk3/1
  cfblk5/1 -> cfblk2/1
  cfblk10/1 -> cfblk6/1
  cfblk6/1 -> cfblk7/1
  cfblk13/1 -> cfblk5/1
  cfblk15/1 -> cfblk9/1
  cfblk8/1 -> cfblk4/1
  cfblk3/1 -> cfblk8/1

== system sampleModel541_pp_difftest/cfblk35/cfblk13 ==
  cfblk1 : Inport
  cfblk10 : Inport  Port=2
  cfblk11 : Inport  Port=3
  cfblk3 : simulink/Discrete/Tapped Delay  vinit=0.0  samptime=-1  NumDelays=1  DelayOrder=Oldest  includeCurrent=off
  cfblk4 : simulink/Discrete/Transfer Fcn Lead or Lag  PoleZ=0.95  ZeroZ=0.75  ICPrevOutput=0.0  ICPrevInput=0.0  DoSatur=off
      settings: SourceProductBaseCode=SL
  cfblk5 : Bias  Bias=[-153657995.643445]
  cfblk6 : simulink/Math Operations/Slider Gain  gain=1  low=0  high=2
  cfblk7 : Polyval  Coefs=[ +2.081618890e-019, -1.441693666e-014, +4.719686976e-010, -8.536869453e-006, +1.621573104e-001, -8.087801117e+001 ]
  cfblk8 : UnaryMinus
  cfblk9 : Constant  Value=[-593567410.518825]  SampleTime=1
  cfblk2 : Outport
  cfblk12 : Outport  Port=2
  cfblk13 : Outport  Port=3
  wires:
  cfblk8/1 -> cfblk12/1
  cfblk7/1 -> cfblk4/1
  cfblk11/1 -> cfblk8/1
  cfblk9/1 -> cfblk5/1
  cfblk3/1 -> cfblk6/1
  cfblk5/1 -> cfblk7/1
  cfblk1/1 -> cfblk13/1
  cfblk10/1 -> cfblk3/1
  cfblk4/1 -> cfblk2/1

== system sampleModel541_pp_difftest/cfblk36/cfblk10 ==
  cfblk1 : Inport
  cfblk7 : Inport  Port=2
  cfblk3 : simulink/Discrete/Transfer Fcn Real Zero  ZeroZ=0.75  ICPrevInput=0.0  DoSatur=off
      settings: SourceProductBaseCode=SL
  cfblk4 : Squeeze
  cfblk5 : Sqrt  Operator=rSqrt  AlgorithmType=Newton-Raphson  SaturateOnIntegerOverflow=on
  cfblk6 : Constant  Value=[137942928.658456]  SampleTime=1
  cfblk2 : Outport
  cfblk8 : Outport  Port=2
  wires:
  cfblk3/1 -> cfblk2/1
  cfblk6/1 -> cfblk8/1
  cfblk4/1 -> cfblk3/1
  cfblk7/1 -> cfblk5/1
  cfblk1/1 -> cfblk4/1

== system sampleModel541_pp_difftest/cfblk36/cfblk11 ==
  cfblk1 : Inport
  cfblk6 : Inport  Port=2
  cfblk7 : Inport  Port=3
  cfblk3 : UnitDelay  HasFrameUpgradeWarning=on
  cfblk4 : UnitDelay  HasFrameUpgradeWarning=on
  cfblk5 : simulink/Math Operations/MinMax Running Resettable  Function=min  vinit=0.0
  cfblk2 : Outport
  wires:
  cfblk4/1 -> cfblk5/1
  cfblk3/1 -> cfblk5/2
  cfblk7/1 -> cfblk3/1
  cfblk6/1 -> cfblk2/1
  cfblk1/1 -> cfblk4/1

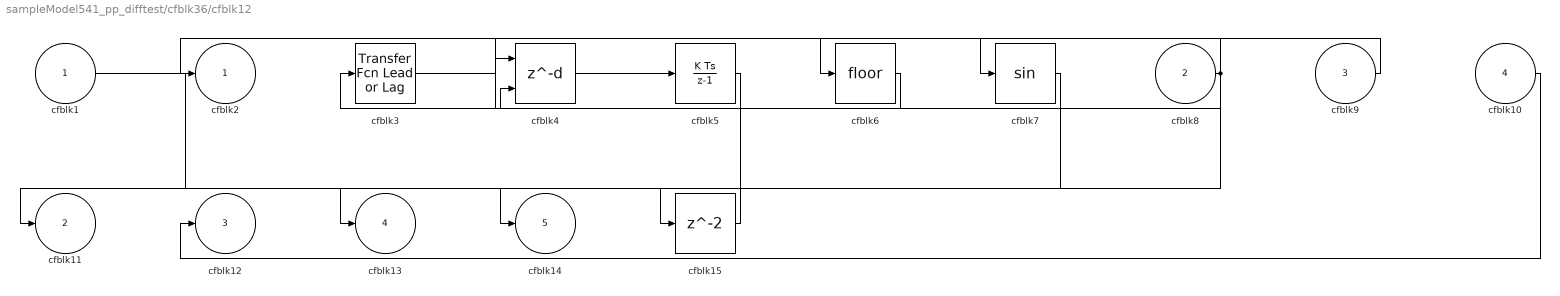
== system sampleModel541_pp_difftest/cfblk36/cfblk12 ==
  cfblk1 : Inport
  cfblk8 : Inport  Port=2
  cfblk9 : Inport  Port=3
  cfblk10 : Inport  Port=4
  cfblk15 : Delay  SampleTime=1
  cfblk3 : simulink/Discrete/Transfer Fcn Lead or Lag  PoleZ=0.95  ZeroZ=0.75  ICPrevOutput=0.0  ICPrevInput=0.0  DoSatur=off
      settings: SourceProductBaseCode=SL
  cfblk4 : Delay  DelayLengthSource=Input port  SampleTime=1
      settings: InputPortMap=u0,p1
  cfblk5 : DiscreteIntegrator  ICPrevOutput=DiscIntNeverNeededParam  ICPrevScaledInput=DiscIntNeverNeededParam
  cfblk6 : Rounding
  cfblk7 : Trigonometry
  cfblk2 : Outport
  cfblk11 : Outport  Port=2
  cfblk12 : Outport  Port=3
  cfblk13 : Outport  Port=4
  cfblk14 : Outport  Port=5
  wires:
  cfblk1/1 -> cfblk13/1
  cfblk10/1 -> cfblk12/1
  cfblk8/1 -> cfblk3/1, cfblk2/1, cfblk11/1
  cfblk9/1 -> cfblk6/1
  cfblk7/1 -> cfblk14/1
  cfblk6/1 -> cfblk4/2
  cfblk4/1 -> cfblk5/1
  cfblk3/1 -> cfblk7/1
  cfblk5/1 -> cfblk15/1
  cfblk15/1 -> cfblk4/1

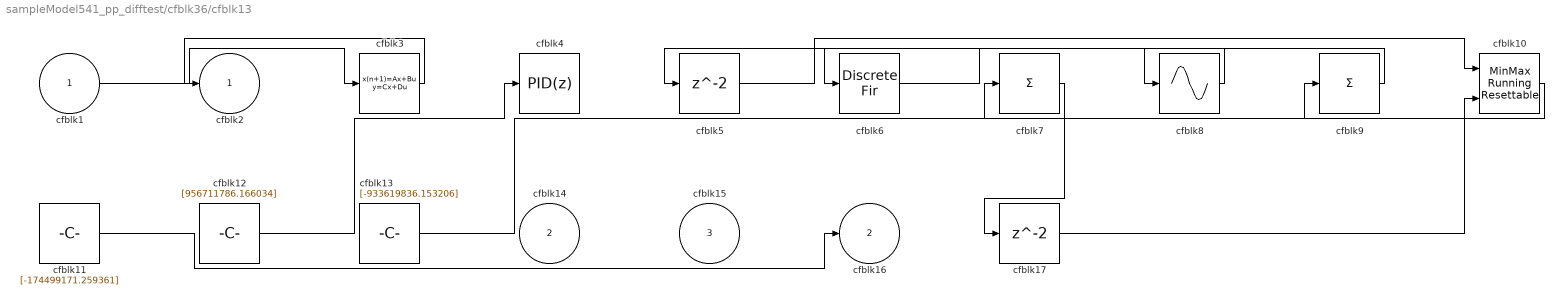
== system sampleModel541_pp_difftest/cfblk36/cfblk13 ==
  cfblk1 : Inport
  cfblk14 : Inport  Port=2
  cfblk15 : Inport  Port=3
  cfblk10 : simulink/Math Operations/MinMax Running Resettable  Function=min  vinit=0.0
  cfblk11 : Constant  Value=[-174499171.259361]  SampleTime=1
  cfblk12 : Constant  Value=[956711786.166034]  SampleTime=1
  cfblk13 : Constant  Value=[-933619836.153206]  SampleTime=1
  cfblk17 : Delay  SampleTime=1
  cfblk3 : DiscreteStateSpace
  cfblk4 : pid_lib/PID Controller  Controller=PID  Form=Parallel  TimeDomain=Discrete-time  UseExternalTs=off  SampleTime=1  IntegratorMethod=Forward Euler  FilterMethod=Forward Euler  ControllerParametersSource=internal  P=1  I=1  D=0  UseFilter=on  N=100  TunerSelectOption=Transfer Function Based (PID Tuner App)  InitialConditionSource=internal  InitialConditionForIntegrator=0  InitialConditionForFilter=0  DifferentiatorICPrevScaledInput=0  ExternalReset=none  TrackingMode=off  Kt=1  LimitOutput=off  SatLimitsSource=internal  UpperSaturationLimit=inf  LowerSaturationLimit=-inf  LinearizeAsGain=off  AntiWindupMode=none  Kb=1  POutMin=[]  POutMax=[]  IOutMin=[]  IOutMax=[]  DOutMin=[]  DOutMax=[]  NOutMin=[]  NOutMax=[]  SumOutMin=[]  SumOutMax=[]  SaturationOutMin=[]  SaturationOutMax=[]  PParamMin=[]  PParamMax=[]  IParamMin=[]  IParamMax=[]  DParamMin=[]  DParamMax=[]  NParamMin=[]  NParamMax=[]  KbParamMin=[]  KbParamMax=[]  KtParamMin=[]  KtParamMax=[]  KbOutMin=[]  KbOutMax=[]  KtOutMin=[]  KtOutMax=[]  IntegratorOutMin=[]  IntegratorOutMax=[]  FilterOutMin=[]  FilterOutMax=[]  SumI1OutMin=[]  SumI1OutMax=[]  SumI2OutMin=[]  SumI2OutMax=[]  SumI3OutMin=[]  SumI3OutMax=[]  SumI4OutMin=[]  SumI4OutMax=[]  SumDOutMin=[]  SumDOutMax=[]  DifferentiatorOutMin=[]  DifferentiatorOutMax=[]  FilterDiffOutCoefMin=[]  FilterDiffOutCoefMax=[]  ReciprocalOutMin=[]  ReciprocalOutMax=[]  SumDenOutMin=[]  SumDenOutMax=[]  SumNumOutMin=[]  SumNumOutMax=[]  DivideOutMin=[]  DivideOutMax=[]  UdiffTsProdOutMin=[]  UdiffTsProdOutMax=[]  NTsProdOutMin=[]  NTsProdOutMax=[]  UintegralTsProdOutMin=[]  UintegralTsProdOutMax=[]  UngainTsProdOutMin=[]  UngainTsProdOutMax=[]  IntegratorContinuousStateAttributes=''  IntegratorStateMustResolveToSignalObject=off  IntegratorRTWStateStorageClass=Auto  FilterContinuousStateAttributes=''  FilterStateMustResolveToSignalObject=off  FilterRTWStateStorageClass=Auto  ParallelPVariant=InternalParameters  IdealPVariant=Disabled  IVariant=InternalParameters  DVariant=InternalParameters  IntegratorVariant=Discrete  SatVariant=Disabled  AWVariant=Passthrough  PCopyVariant=Disabled  TRVariant=Disabled  FdbkBlocksVariant=Forward  IdealPFdbkVariant=Disabled  SatFdbkVariant=Disabled  DerivativeFilterVariant=ForwardEulerFilter  NVariant=InternalParameters  NCopyVariant=Disabled  FilterICVariant=InternalICsFilter  IntegratorICVariant=InternalICs  ExternalResetVariant=Disabled  TRSumVariant=Passthrough  SumFdbkVariant=Disabled  SumVariant=Sum_PID  TsampFilterVariant=InternalTs  TsampNgainVariant=Passthrough  TsampIntegralVariant=Passthrough  ExternalSaturationOutDataTypeStr=Inherit: Same as second input
  cfblk5 : Delay  SampleTime=1
  cfblk6 : DiscreteFir  SampleTime=1
  cfblk7 : Sum  Inputs=+
  cfblk8 : Sin  TimeSource=Use external signal  SampleTime=0
  cfblk9 : Sum  Inputs=+
  cfblk2 : Outport
  cfblk16 : Outport  Port=2
  wires:
  cfblk1/1 -> cfblk3/1
  cfblk9/1 -> cfblk6/1
  cfblk10/1 -> cfblk7/1
  cfblk12/1 -> cfblk4/1
  cfblk3/1 -> cfblk2/1
  cfblk6/1 -> cfblk8/1
  cfblk5/1 -> cfblk10/1
  cfblk13/1 -> cfblk9/1
  cfblk11/1 -> cfblk16/1
  cfblk8/1 -> cfblk5/1
  cfblk7/1 -> cfblk17/1
  cfblk17/1 -> cfblk10/2
